simulink model "WaveGeneration"  (R2025a)
settings: Solver=VariableStepAuto  StartTime=0.0  StopTime=10.0  RelTol=1e-3
undefined symbols (not defined in the file): PWM_FREQ, TS
libraries: eeGeneralControl x1, simulink x1
settings Model: DataDictionary=PwmGenerator.sldd  Creator=tecnicomcbti  LastModifiedBy=tecnicomcbti

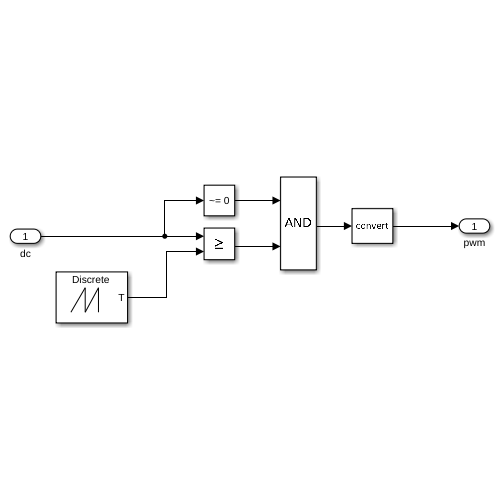
[thumbnail: Simulink's stored preview of the top-level diagram]
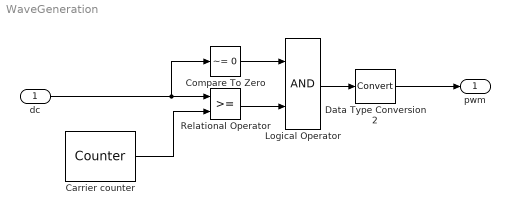
== system WaveGeneration ==
  dc : Inport  SampleTime=TS
  Carrier counter : eeGeneralControl/Counter  CarrCount=Up  Range=[0 1]  Tper=1/PWM_FREQ  Tdelay=T_DELAY  Ts=TS
  Compare To Zero : simulink/Logic and Bit Operations/Compare To Zero  relop=~=  OutDataTypeStr=boolean
  Data Type Conversion2 : DataTypeConversion  SaturateOnIntegerOverflow=off  RndMeth=Floor
  Logical Operator : Logic  AllPortsSameDT=off  OutDataTypeStr=boolean
  Relational Operator : RelationalOperator  OutDataTypeStr=boolean  RndMeth=Simplest  InputSameDT=off
  pwm : Outport  VectorParamsAs1DForOutWhenUnconnected=off
  wires:
  Compare To Zero/1 -> Logical Operator/1
  Logical Operator/1 -> Data Type Conversion2/1
  Data Type Conversion2/1 -> pwm/1
  Carrier counter/1 -> Relational Operator/2
  Relational Operator/1 -> Logical Operator/2
  dc/1 -> Compare To Zero/1, Relational Operator/1
